simulink model "QDrone_IO_Check_Full_r2018a"  (Simulink 9.1)
settings: Solver=ode2  StartTime=0.0  StopTime=inf  FixedStep=0.001  RelTol=1e-3  EnableMultiTasking=on
model workspace (MAT data in the model file):
  Sig = Simulink.Signal
  Sig.DataType = 'auto'
  Sig.Dimensions = -1
  Sig.DimensionsMode = 'auto'
  Sig.Complexity = 'auto'
  Sig.SampleTime = -1
  Sig.SamplingMode = 'auto'
  video_step_size = 0.06
InitFcn:
  | set_param('QDrone_IO_Check_Full/Motor Switch', 'sw', '0');
undefined symbols (not defined in the file): HIL, qc_get_step_size
libraries: quarc_library x26, simulink x8, simulink_extras x3
settings Model: Creator=Admin  LastModifiedBy=user  SimulationMode=external
settings SolverCC: PositivePriorityOrder=on
settings DataIOCC: SaveFormat=Dataset
settings OptimizationCC: LifeSpan=auto
settings DebuggingCC: UnderspecifiedInitializationDetection=Simplified  MergeDetectMultiDrivingBlocksExec=error  ParameterPrecisionLossMsg=none
settings HardwareCC: ProdBitPerLong=64  ProdBitPerPointer=64  ProdBitPerSizeT=64  ProdBitPerPtrDiffT=64  ProdLargestAtomicFloat=Float  ProdIntDivRoundTo=Zero  ProdEndianess=LittleEndian  ProdWordSize=64  ProdHWDeviceType=Intel->x86-64 (Linux 64)
settings ModelReferenceCC: PropagateSignalLabelsOutOfModel=on
settings RTWCC: Description=QUARC Linux x64 Target (QDrone) Using Toolchain  SystemTargetFile=quarc_linux_x64.tlc  TemplateMakefile=quarc_default_tmf  Toolchain=QUARC linux_x64 | gmake (64-bit Windows)  BuildConfiguration=Faster Runs
settings STFCustomTargetCC: ConcurrentExecutionCompliant=on  UseToolchainInfoCompliant=on  SystemTargetFile=quarc_linux_x64.tlc
settings GRTTargetCC: ParMdlRefBuildCompliant=off  CompOptLevelCompliant=off  MatFileLogging=off  CPPClassGenCompliant=off  ExtMode=on  ExtModeMexFile=quarc_comm  ExtModeMexArgs='-w -d /tmp -uri %u','tcpip://QDrone0xxxxx.local:17001'

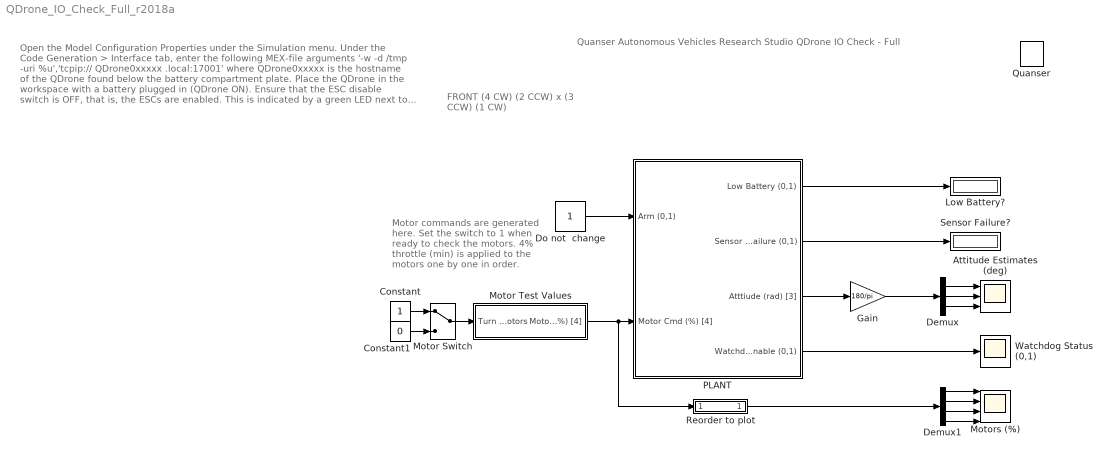
== system QDrone_IO_Check_Full_r2018a ==
  note: FRONT
      |
      | (4 CW)           (2 CCW)
      |
      |                 x
      |
      | (3 CCW)        (1 CW)
  note: Motor commands are generated here.
      |
      | Set the switch to 1 when ready to check
      | the motors. 4% throttle (min) is applied
      | to the motors one by one in order.
  note: Quanser Autonomous Vehicles Research Studio
      | QDrone IO Check - Full
  note: Open the Model Configuration Properties under the Simulation menu.
      |
      | Under the Code Generation > Interface tab, enter the following MEX-file arguments
      |
      | '-w -d /tmp -uri %u','tcpip:// QDrone0xxxxx .local:17001'
      |
      | where QDrone0xxxxx is the hostname of the QDrone found below the battery compartment plate.
      |
      | Place the QDrone in the workspace with a battery plugged in (QDrone ON).
      |
      | Ensure that the ESC disable switch is OFF, that is, the ESCs are enabled. This is indicated by a green LED next to the switch.
      |
      | Ensure that a connection to the drone is established by pinging to it. See the Research Studio Setup documentation (the Communicating with the QDrone section).
      |
      | Under the QUARC menu, click on Build .
      |
      | Ensure that the Motor Switch is set to 0 in this model.
      |
      | Under the QUARC menu, click on Start .
      |
      | After you hear 2 beeps (which indicates that the model has started running on the QDrone and that the ESCs are ENABLED), set the Motor Switch to 1.
      |
      | Ensure that the motors are spinning in order and directions specified in the Motors scope (they should turn on in the order of a clockwise circle).
      |
      | Set the Motor Switch to 0. Enter the workspace and set the ESC disable switch ON. This is indicated by a red LED next to the switch.
      |
      | Move the drone manually. Check the attitude of the drone in the Attitude Estimates (deg) scope to ensure that the readings are reasonable.
      | NOTE : Hold the drone using the handle on the top frame of the drone
      | NOTE : DO NOT handle the drone with spinning motors.
      | NOTE : Ensure that the motors are not spinning (Motor Switch set to 0). It is dangerous to handle the drone with spinning motors.
      |
      | Ensure that the Low Battery display shows 0 (as in your new Battery is not low. The low battery threshold is set to 10.5V)
      |
      | Ensure that the Sensor display shows 0 (no sensor failure detected).
  Attitude Estimates (deg) : Scope  NumInputPorts=3
  Constant : Constant
  Constant1 : Constant  Value=0
  Demux : Demux  Outputs=3
  Demux1 : Demux
  Do not  change : Constant
  Gain : Gain  Gain=180/pi
  Low Battery? : Display
      settings: Decimation=100
  Motor Switch : ManualSwitch
  Motor Test Values : Subsystem
  Motors (%) : Scope  NumInputPorts=4
  PLANT : Subsystem
  Quanser : quarc_library/Logos/Quanser
  Reorder to plot : Subsystem
  Sensor Failure? : Display
      settings: Decimation=100
  Watchdog Status (0,1) : Scope
  wires:
  PLANT/3(Atttiude (rad) [3]) -> Gain/1
  Constant/1 -> Motor Switch/1
  Constant1/1 -> Motor Switch/2
  Motor Test Values/1(Motor Cmd (%) [4]) -> Reorder to plot/1(" "), PLANT/2(Motor Cmd (%) [4])
  Demux1/1 -> Motors (%)/1
  Demux1/2 -> Motors (%)/2
  Demux1/3 -> Motors (%)/3
  Demux1/4 -> Motors (%)/4
  Demux/1 -> Attitude Estimates (deg)/1
  Demux/2 -> Attitude Estimates (deg)/2
  Demux/3 -> Attitude Estimates (deg)/3
  Motor Switch/1 -> Motor Test Values/1(Turn Motors)
  Gain/1 -> Demux/1
  Reorder to plot/1("  ") -> Demux1/1
  PLANT/2(Sensor Failure (0,1)) -> Sensor Failure?/1
  Do not  change/1 -> PLANT/1(Arm (0,1))
  PLANT/1(Low Battery (0,1)) -> Low Battery?/1
  PLANT/4(Watchdog Enable (0,1)) -> Watchdog Status (0,1)/1

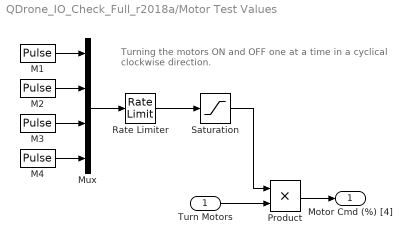
== system QDrone_IO_Check_Full_r2018a/Motor Test Values ==
  note: Turning the motors ON and OFF one at a time in a cyclical
      | clockwise direction.
  Turn Motors : Inport
  M1 : DiscretePulseGenerator  PulseType=Time based  Amplitude=0.04  Period=8  PulseWidth=12.5
  M2 : DiscretePulseGenerator  PulseType=Time based  Amplitude=0.04  Period=8  PulseWidth=12.5  PhaseDelay=6
  M3 : DiscretePulseGenerator  PulseType=Time based  Amplitude=0.04  Period=8  PulseWidth=12.5  PhaseDelay=2
  M4 : DiscretePulseGenerator  PulseType=Time based  Amplitude=0.04  Period=8  PulseWidth=12.5  PhaseDelay=4
  Mux : Mux
  Product : Product
  Rate Limiter : RateLimiter  RisingSlewLimit=0.1  FallingSlewLimit=-0.1  SampleTimeMode=inherited
  Saturation : Saturate  UpperLimit=0.1  LowerLimit=0
  Motor Cmd (%) [4] : Outport  VectorParamsAs1DForOutWhenUnconnected=off
  wires:
  M2/1 -> Mux/2
  M3/1 -> Mux/3
  M4/1 -> Mux/4
  M1/1 -> Mux/1
  Mux/1 -> Rate Limiter/1
  Rate Limiter/1 -> Saturation/1
  Saturation/1 -> Product/1
  Product/1 -> Motor Cmd (%) [4]/1
  Turn Motors/1 -> Product/2

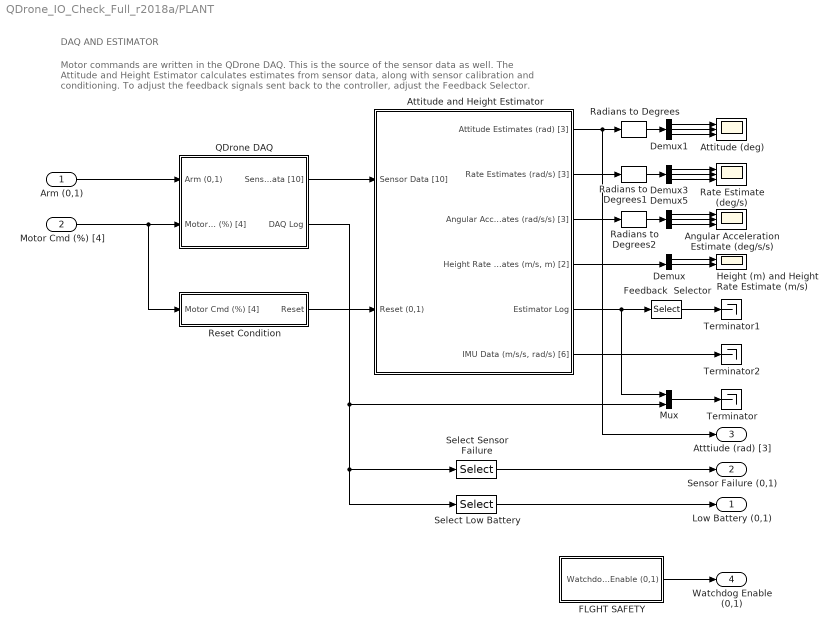
== system QDrone_IO_Check_Full_r2018a/PLANT ==
  note: Motor commands are written in the QDrone DAQ. This is the source of the sensor data as well. The Attitude and Height Estimator calculates estimates from sensor data, along with sensor calibration and conditioning. To adjust the feedback signals sent back to the controller, adjust the Feedback Selector.
  note: DAQ AND ESTIMATOR
  Arm (0,1) : Inport
  Motor Cmd (%) [4] : Inport  Port=2
  Angular Acceleration Estimate (deg/s/s) : Scope  NumInputPorts=3
  Attitude (deg) : Scope  NumInputPorts=3
  Attitude and Height Estimator : Subsystem
  Demux : Demux  Outputs=2
  Demux1 : Demux  Outputs=3
  Demux3 : Demux  Outputs=3
  Demux5 : Demux  Outputs=3
  FLGHT SAFETY : Subsystem
  Feedback  Selector : Selector  InputPortWidth=11  IndexOptions=Index vector (dialog)  Indices=[1:9]  OutputSizes=1
  Height (m) and Height Rate Estimate (m/s) : Scope  NumInputPorts=2
  Mux : Mux  Inputs=[11 13]
  QDrone DAQ : Subsystem
  Radians to Degrees : simulink_extras/Transformations/Radians to Degrees
  Radians to Degrees1 : simulink_extras/Transformations/Radians to Degrees
  Radians to Degrees2 : simulink_extras/Transformations/Radians to Degrees
  Rate Estimate (deg/s) : Scope  NumInputPorts=3
  Reset Condition : Subsystem
  Select Low Battery : Selector  InputPortWidth=13  IndexOptions=Index vector (dialog)  Indices=[3]  OutputSizes=1
  Select Sensor Failure : Selector  InputPortWidth=13  IndexOptions=Index vector (dialog)  Indices=[1]  OutputSizes=1
  Terminator : Terminator
  Terminator1 : Terminator
  Terminator2 : Terminator
  Low Battery (0,1) : Outport  VectorParamsAs1DForOutWhenUnconnected=off
  Sensor Failure (0,1) : Outport  Port=2  VectorParamsAs1DForOutWhenUnconnected=off
  Atttiude (rad) [3] : Outport  Port=3  VectorParamsAs1DForOutWhenUnconnected=off
  Watchdog Enable (0,1) : Outport  Port=4  VectorParamsAs1DForOutWhenUnconnected=off
  wires:
  Mux/1 -> Terminator/1
  QDrone DAQ/1(Sensor Data [10]) -> Attitude and Height Estimator/1(Sensor Data [10])
  Attitude and Height Estimator/4("Height Rate and  Height Estimates (m/s, m) [2]") -> Demux/1
  Attitude and Height Estimator/1(Attitude Estimates (rad) [3]) -> Atttiude (rad) [3]/1, Radians to Degrees/1
  Demux1/1 -> Attitude (deg)/1
  Demux1/2 -> Attitude (deg)/2
  Demux1/3 -> Attitude (deg)/3
  Demux3/1 -> Rate Estimate (deg/s)/1
  Demux3/2 -> Rate Estimate (deg/s)/2
  Demux3/3 -> Rate Estimate (deg/s)/3
  Demux5/1 -> Angular Acceleration Estimate (deg/s/s)/1
  Demux5/2 -> Angular Acceleration Estimate (deg/s/s)/2
  Demux5/3 -> Angular Acceleration Estimate (deg/s/s)/3
  Attitude and Height Estimator/2(Rate Estimates (rad/s) [3]) -> Radians to Degrees1/1
  Attitude and Height Estimator/3(Angular Acceleration Estimates (rad/s/s) [3]) -> Radians to Degrees2/1
  Demux/2 -> Height (m) and Height Rate Estimate (m/s)/2
  Demux/1 -> Height (m) and Height Rate Estimate (m/s)/1
  Attitude and Height Estimator/5(Estimator Log) -> Feedback  Selector/1, Mux/1
  Reset Condition/1(Reset) -> Attitude and Height Estimator/2(Reset (0,1))
  Motor Cmd (%) [4]/1 -> QDrone DAQ/2(Motor Cmd (%) [4]), Reset Condition/1(Motor Cmd (%) [4])
  Arm (0,1)/1 -> QDrone DAQ/1(Arm (0,1))
  Feedback  Selector/1 -> Terminator1/1
  QDrone DAQ/2(DAQ Log) -> Select Sensor Failure/1, Select Low Battery/1, Mux/2
  Select Low Battery/1 -> Low Battery (0,1)/1
  Select Sensor Failure/1 -> Sensor Failure (0,1)/1
  Attitude and Height Estimator/6("IMU Data (m/s/s, rad/s) [6]") -> Terminator2/1
  Radians to Degrees/1 -> Demux1/1
  Radians to Degrees1/1 -> Demux3/1
  Radians to Degrees2/1 -> Demux5/1
  FLGHT SAFETY/1(Watchdog Enable (0,1)) -> Watchdog Enable (0,1)/1

== system QDrone_IO_Check_Full_r2018a/Reorder to plot ==
  " " : Inport
  Demux : Demux
  Mux : Mux
  "  " : Outport  VectorParamsAs1DForOutWhenUnconnected=off
  wires:
  Demux/3 -> Mux/2
  Demux/4 -> Mux/1
  Mux/1 -> "  "/1
  Demux/2 -> Mux/3
  Demux/1 -> Mux/4
  " "/1 -> Demux/1

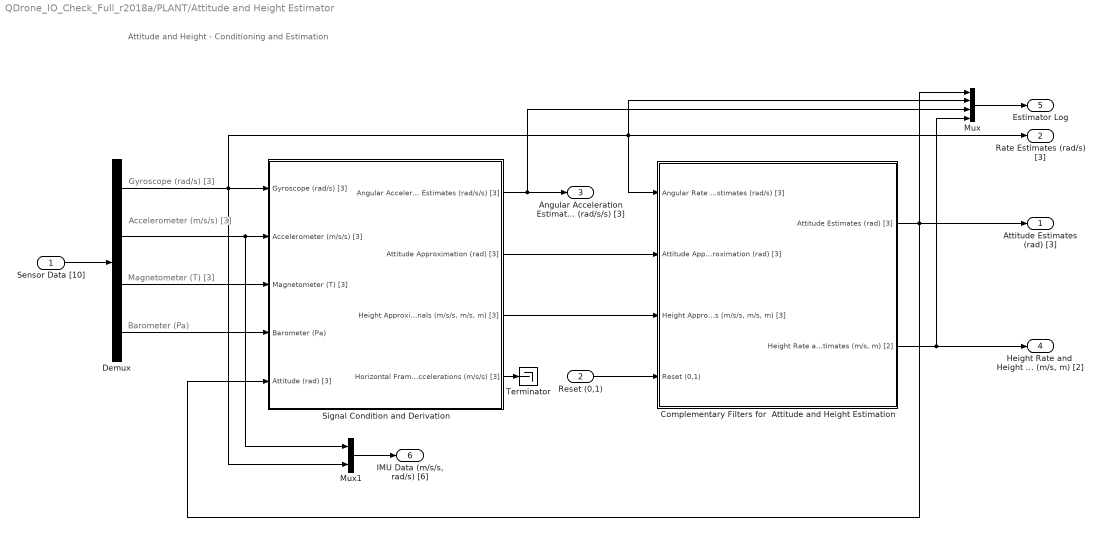
== system QDrone_IO_Check_Full_r2018a/PLANT/Attitude and Height Estimator ==
  note: Attitude and Height - Conditioning and Estimation
  note: Gyroscope (rad/s) [3]
  note: Accelerometer (m/s/s) [3]
  note: Magnetometer (T) [3]
  note: Barometer (Pa)
  Sensor Data [10] : Inport
  Reset (0,1) : Inport  Port=2
  Complementary Filters for  Attitude and Height Estimation : Subsystem
  Demux : Demux  Outputs=[3 3 3 1]
  Mux : Mux  Inputs=[3 3 3 2]
  Mux1 : Mux  Inputs=2
  Signal Condition and Derivation : Subsystem
  Terminator : Terminator
  Attitude Estimates (rad) [3] : Outport  VectorParamsAs1DForOutWhenUnconnected=off
  Rate Estimates (rad/s) [3] : Outport  Port=2  VectorParamsAs1DForOutWhenUnconnected=off
  Angular Acceleration Estimates (rad/s/s) [3] : Outport  Port=3  VectorParamsAs1DForOutWhenUnconnected=off
  "Height Rate and  Height Estimates (m/s, m) [2]" : Outport  Port=4  VectorParamsAs1DForOutWhenUnconnected=off
  Estimator Log : Outport  Port=5  VectorParamsAs1DForOutWhenUnconnected=off
  "IMU Data (m/s/s, rad/s) [6]" : Outport  Port=6  VectorParamsAs1DForOutWhenUnconnected=off
  wires:
  Complementary Filters for  Attitude and Height Estimation/2("Height Rate and  Height Estimates (m/s, m) [2]") -> "Height Rate and  Height Estimates (m/s, m) [2]"/1, Mux/4
  Signal Condition and Derivation/2(Attitude Approximation (rad) [3]) -> Complementary Filters for  Attitude and Height Estimation/2(Attitude Approximation (rad) [3])
  Signal Condition and Derivation/3("Height Approximation Signals (m/s/s, m/s, m) [3]") -> Complementary Filters for  Attitude and Height Estimation/3("Height Approximation Signals (m/s/s, m/s, m) [3]")
  Demux/2 -> Mux1/1, Signal Condition and Derivation/2(Accelerometer (m/s/s) [3])
  Demux/3 -> Signal Condition and Derivation/3(Magnetometer (T) [3])
  Demux/4 -> Signal Condition and Derivation/4(Barometer (Pa))
  Sensor Data [10]/1 -> Demux/1
  Mux/1 -> Estimator Log/1
  Reset (0,1)/1 -> Complementary Filters for  Attitude and Height Estimation/4(Reset (0,1))
  Complementary Filters for  Attitude and Height Estimation/1(Attitude Estimates (rad) [3]) -> Attitude Estimates (rad) [3]/1, Signal Condition and Derivation/5(Attitude (rad) [3]), Mux/1
  Signal Condition and Derivation/1(Angular Acceleration Estimates (rad/s/s) [3]) -> Mux/3, Angular Acceleration Estimates (rad/s/s) [3]/1
  Demux/1 -> Rate Estimates (rad/s) [3]/1, Mux/2, Complementary Filters for  Attitude and Height Estimation/1(Angular Rate Estimates (rad/s) [3]), Mux1/2, Signal Condition and Derivation/1(Gyroscope (rad/s) [3])
  Mux1/1 -> "IMU Data (m/s/s, rad/s) [6]"/1
  Signal Condition and Derivation/4(Horizontal Frame Accelerations (m/s/s) [3]) -> Terminator/1

== system QDrone_IO_Check_Full_r2018a/PLANT/FLGHT SAFETY ==
  note: Show if the watchdog is enabled/disabled via ESC enable switch.
  Data Type Conversion : DataTypeConversion  OutDataTypeStr=boolean
  HIL Watchdog : quarc_library/Data Acquisition/Generic/Watchdog/HIL Watchdog  object_name=HIL-1  timeout=0.1  sample_time=qc_get_step_size  active=off
      settings: AttributesFormatString=(%<object_name>)  SourceProductName=QUARC Targets
  Watchdog Enable (0,1) : Outport  VectorParamsAs1DForOutWhenUnconnected=off
  wires:
  HIL Watchdog/1 -> Data Type Conversion/1
  Data Type Conversion/1 -> Watchdog Enable (0,1)/1

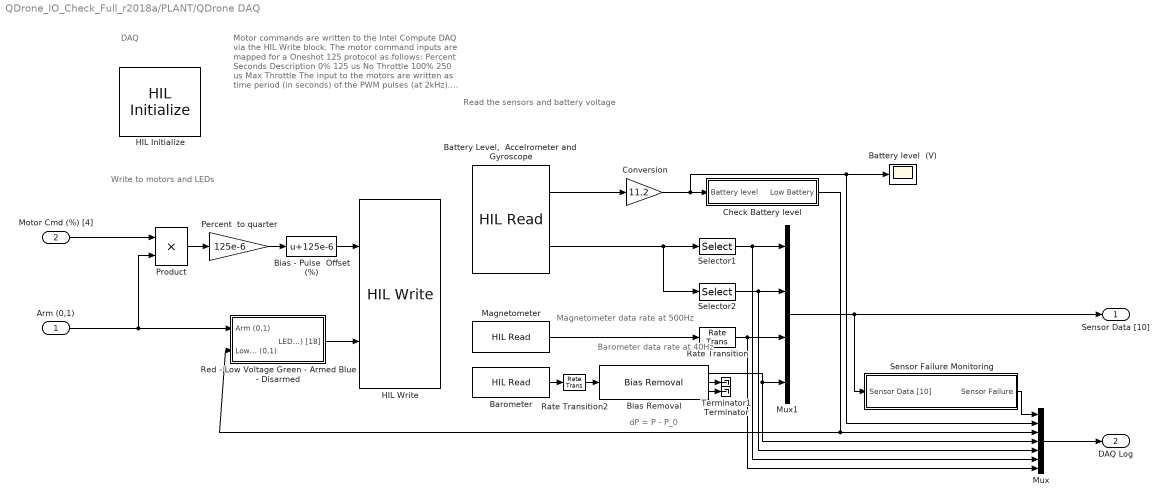
== system QDrone_IO_Check_Full_r2018a/PLANT/QDrone DAQ ==
  note: Read the sensors and battery voltage
  note: Write to motors and LEDs
  note: DAQ
  note: Motor commands are written to the Intel Compute DAQ via the HIL Write block. The motor command inputs are mapped for a Oneshot 125 protocol as follows:
      |
      | Percent Seconds Description
      | 0% 125 us No Throttle
      | 100% 250 us Max Throttle
      |
      | The input to the motors are written as time period (in seconds) of the PWM pulses (at 2kHz).
      |
      | LED colors can be set using a simple 3x1 ON (1) and OFF (0) vector (RGB mode).
  note: Barometer data rate at 40Hz
  note: Magnetometer data rate at 500Hz
  note: dP = P - P_0
  Arm (0,1) : Inport
  Motor Cmd (%) [4] : Inport  Port=2
  Barometer : quarc_library/Data Acquisition/Generic/Immediate I//O/HIL Read  Priority=1  object_name=HIL-1  analog_channels=[]  encoder_channels=[]  digital_channels=[]  other_channels=[9000]  sample_time=qc_get_step_size*25  active=on  vector_output=on  data_type_mode=Inherit via back propagation  encoder_data_type=double  digital_data_type=boolean
      settings: SourceProductName=The database C:\Users\user\AppData\Roaming\MathWorks\MATLAB\R2017a\slblocks_master.db is locked, or a table in the database is locked. (database is locked)
  "Battery Level,  Accelrometer and  Gyroscope" : quarc_library/Data Acquisition/Generic/Immediate I//O/HIL Read  Priority=1  object_name=HIL-1  analog_channels=[4]  encoder_channels=[]  digital_channels=[]  other_channels=[3000:3002 4000:4002]  sample_time=qc_get_step_size  active=on  vector_output=on  data_type_mode=Inherit via back propagation  encoder_data_type=double  digital_data_type=boolean
      settings: SourceProductName=The database C:\Users\user\AppData\Roaming\MathWorks\MATLAB\R2017a\slblocks_master.db is locked, or a table in the database is locked. (database is locked)
  Battery level  (V) : Scope
  Bias - Pulse  Offset (%) : Bias  Bias=125e-6
  Bias Removal : quarc_library/Discrete/Bias Removal  start_time=0  end_time=2  switch_id=X  sample_time=qc_get_step_size
      settings: SourceProductName=QUARC Targets
  Check Battery level : Subsystem
  Conversion : Gain  Gain=11.2
  HIL Initialize : quarc_library/Data Acquisition/Generic/Configuration/HIL Initialize  object_name=HIL-1  board_type=qdrone  board_number=0  board_options=gyro_fs=2000;gyro_rate=1000;gyro_os=4;accel_fs=16;accel_rate=400;accel_os=4;baro_os=4096  exclusive=off  active=on  hardware_clocks=[]  clock_modes=[]  initial_clock_frequencies=[]  set_clock_params_at_start=off  set_clock_params_at_switch_in=off  set_clock_frequencies_at_start=off  set_clock_frequencies_at_switch_in=off  analog_input_channels=[0:4]  analog_input_configurations=[]  analog_input_maximums=[3.3]  analog_input_minimums=[0]  set_analog_input_params_at_start=off  set_analog_input_params_at_switch_in=off  analog_output_channels=[]  analog_output_maximums=[]  analog_output_minimums=[]  initial_analog_outputs=[]  final_analog_outputs=[]  watchdog_analog_outputs=[]  set_analog_output_params_at_start=off  set_analog_output_params_at_switch_in=off  set_analog_outputs_at_start=off  set_analog_outputs_at_switch_in=off  set_analog_outputs_at_terminate=off  set_analog_outputs_at_switch_out=off  set_analog_outputs_on_watchdog=off  digital_input_channels=[]  digital_output_channels=[5:7 9:23]  digital_output_configuration=[]  initial_digital_outputs=[0]  final_digital_outputs=[0]  watchdog_digital_outputs=[]  set_digital_output_params_at_start=off  set_digital_output_params_at_switch_in=off  set_digital_outputs_at_start=on  set_digital_outputs_at_switch_in=off  set_digital_outputs_at_terminate=on  set_digital_outputs_at_switch_out=off  set_digital_outputs_on_watchdog=off  encoder_channels=[0:2]  quadrature=[4]  encoder_filter_frequency=50e6/1  initial_encoder_counts=[0]  set_encoder_params_at_start=on  set_encoder_params_at_switch_in=off  set_encoder_counts_at_start=on  set_encoder_counts_at_switch_in=off  pwm_channels=[0:3]  pwm_modes=[4]  pwm_frequency=2000  pwm_configuration=[0]  pwm_alignment=[0]  pwm_polarity=[1]  pwm_leading_deadband=[]  pwm_trailing_deadband=[]  initial_pwm_outputs=[0]  final_pwm_outputs=[0]  watchdog_pwm_outputs=[0]  set_pwm_params_at_start=on  set_pwm_params_at_switch_in=off  set_pwm_outputs_at_start=on  set_pwm_outputs_at_switch_in=off  set_pwm_outputs_at_terminate=on  set_pwm_outputs_at_switch_out=off  set_pwm_outputs_on_watchdog=off  other_output_channels=[]  initial_other_outputs=[]  final_other_outputs=[]  watchdog_other_outputs=[]  set_other_outputs_at_start=off  set_other_outputs_at_switch_in=off  set_other_outputs_at_terminate=off  set_other_outputs_at_switch_out=off  set_other_outputs_on_watchdog=off
      settings: SourceProductName=The database C:\Users\user\AppData\Roaming\MathWorks\MATLAB\R2017a\slblocks_master.db is locked, or a table in the database is locked. (database is locked)
  HIL Write : quarc_library/Data Acquisition/Generic/Immediate I//O/HIL Write  object_name=HIL-1  analog_channels=[]  pwm_channels=[0:3]  digital_channels=[5:7 9:23]  other_channels=[]  sample_time=-1  active=off  vector_input=on
      settings: SourceProductName=The database C:\Users\user\AppData\Roaming\MathWorks\MATLAB\R2017a\slblocks_master.db is locked, or a table in the database is locked. (database is locked)
  Magnetometer : quarc_library/Data Acquisition/Generic/Immediate I//O/HIL Read  Priority=1  object_name=HIL-1  analog_channels=[]  encoder_channels=[]  digital_channels=[]  other_channels=[8000:8002]  sample_time=qc_get_step_size*2  active=on  vector_output=on  data_type_mode=Inherit via back propagation  encoder_data_type=double  digital_data_type=boolean
      settings: SourceProductName=The database C:\Users\user\AppData\Roaming\MathWorks\MATLAB\R2017a\slblocks_master.db is locked, or a table in the database is locked. (database is locked)
  Mux : Mux  Inputs=[1 1 1 1 3 3 3]
  Mux1 : Mux  Inputs=[3 3 3 1]
  Percent  to quarter : Gain  Gain=125e-6
  Product : Product
  Rate Transition : RateTransition
  Rate Transition2 : RateTransition  OutPortSampleTime=qc_get_step_size
  Red - Low Voltage Green - Armed Blue - Disarmed : Subsystem
  Selector1 : Selector  InputPortWidth=6  IndexOptions=Index vector (dialog)  Indices=[1:3]  OutputSizes=1
  Selector2 : Selector  InputPortWidth=6  IndexOptions=Index vector (dialog)  Indices=[4:6]  OutputSizes=1
  Sensor Failure Monitoring : Subsystem
  Terminator : Terminator
  Terminator1 : Terminator
  Sensor Data [10] : Outport  VectorParamsAs1DForOutWhenUnconnected=off
  DAQ Log : Outport  Port=2  VectorParamsAs1DForOutWhenUnconnected=off
  wires:
  Percent  to quarter/1 -> Bias - Pulse  Offset (%)/1
  Arm (0,1)/1 -> Product/2, Red - Low Voltage Green - Armed Blue - Disarmed/1(Arm (0,1))
  "Battery Level,  Accelrometer and  Gyroscope"/2 -> Selector2/1, Selector1/1
  Check Battery level/1(Low Battery) -> Mux/3, Red - Low Voltage Green - Armed Blue - Disarmed/2(Low Battery (0,1))
  Sensor Failure Monitoring/1(Sensor Failure) -> Mux/1
  Magnetometer/1 -> Rate Transition/1
  Mux/1 -> DAQ Log/1
  Bias Removal/1 -> Mux/4, Mux1/4
  Selector2/1 -> Mux/5, Mux1/2
  Selector1/1 -> Mux/6, Mux1/1
  Rate Transition/1 -> Mux/7, Mux1/3
  "Battery Level,  Accelrometer and  Gyroscope"/1 -> Conversion/1
  Mux1/1 -> Sensor Data [10]/1, Sensor Failure Monitoring/1(Sensor Data [10])
  Motor Cmd (%) [4]/1 -> Product/1
  Conversion/1 -> Battery level  (V)/1, Mux/2, Check Battery level/1(Battery level)
  Bias - Pulse  Offset (%)/1 -> HIL Write/1
  Red - Low Voltage Green - Armed Blue - Disarmed/1(LEDs (%) [18]) -> HIL Write/2
  Product/1 -> Percent  to quarter/1
  Bias Removal/3 -> Terminator/1
  Bias Removal/2 -> Terminator1/1
  Barometer/1 -> Rate Transition2/1
  Rate Transition2/1 -> Bias Removal/1

== system QDrone_IO_Check_Full_r2018a/PLANT/Reset Condition ==
  note: Detect motor start condition and reset estimators.
      | Default threshold is if motor commands are greater than minimum throttle (5% of max.) for over 0.2 seconds.
  Motor Cmd (%) [4] : Inport
  Compare : quarc_library/Logic Operations/Compare  operator=>  output_data_type=boolean
      settings: SourceProductName=QUARC Targets
  For some time continuously : quarc_library/Discontinuities/Threshold  operator=>=  param_src=Specify via dialog  threshold=0.5  duration=0.2
      settings: SourceProductName=QUARC Targets
  Logical Operator : Logic  Inputs=1  AllPortsSameDT=off  OutDataTypeStr=boolean
  Minimum Throttle (%) : Constant  Value=[0.05 0.05 0.05 0.05]
  Terminator4 : Terminator
  Reset : Outport  VectorParamsAs1DForOutWhenUnconnected=off
  wires:
  For some time continuously/1 -> Reset/1
  Motor Cmd (%) [4]/1 -> Compare/1
  For some time continuously/2 -> Terminator4/1
  Compare/1 -> Logical Operator/1
  Minimum Throttle (%)/1 -> Compare/2
  Logical Operator/1 -> For some time continuously/1

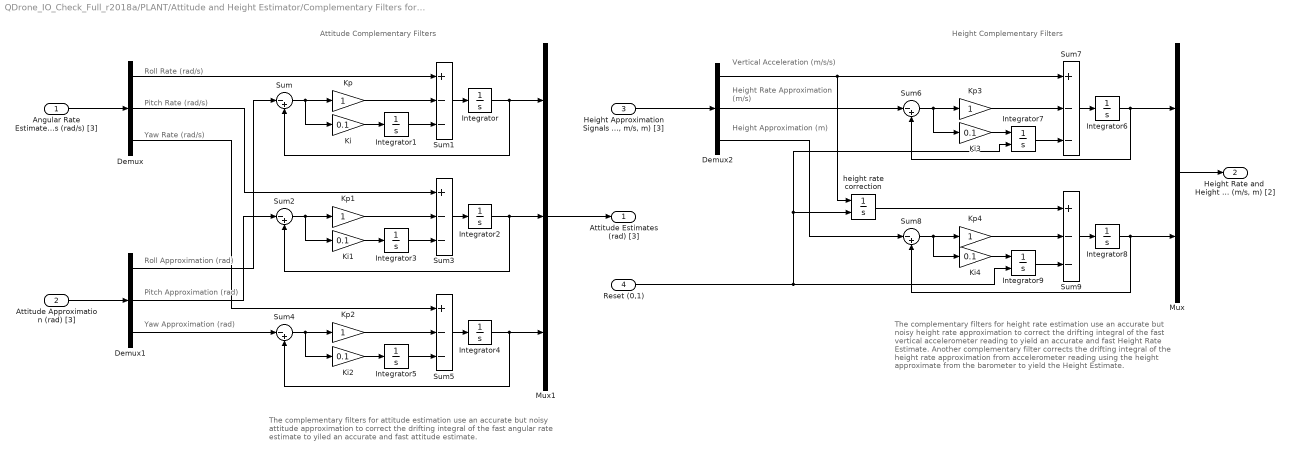
== system QDrone_IO_Check_Full_r2018a/PLANT/Attitude and Height Estimator/Complementary Filters for  Attitude and Height Estimation ==
  note: Attitude Complementary Filters
  note: The complementary filters for attitude estimation use an accurate but noisy attitude approximation to correct the drifting integral of the fast angular rate estimate to yiled an accurate and fast attitude estimate.
  note: Roll Rate (rad/s)
  note: Pitch Rate (rad/s)
  note: Yaw Rate (rad/s)
  note: Roll Approximation (rad)
  note: Pitch Approximation (rad)
  note: Yaw Approximation (rad)
  note: Height Rate Approximation (m/s)
  note: Height Approximation (m)
  note: Vertical Acceleration (m/s/s)
  note: Height Complementary Filters
  note: The complementary filters for height rate estimation use an accurate but noisy height rate approximation to correct the drifting integral of the fast vertical accelerometer reading to yield an accurate and fast Height Rate Estimate. Another complementary filter corrects the drifting integral of the height rate approximation from accelerometer reading using the height approximate from the barometer to yield the Height Estimate.
  Angular Rate Estimates (rad/s) [3] : Inport
  Attitude Approximation (rad) [3] : Inport  Port=2
  "Height Approximation Signals (m/s/s, m/s, m) [3]" : Inport  Port=3
  Reset (0,1) : Inport  Port=4
  Demux : Demux  Outputs=3
  Demux1 : Demux  Outputs=3
  Demux2 : Demux  Outputs=3
  Integrator{,1..6,8} (8 alike) : Integrator
  Integrator7 : Integrator  ExternalReset=rising
  Integrator9 : Integrator  ExternalReset=rising
  Ki{,1..4} (5 alike) : Gain  Gain=0.1
  Kp{,1..4} (5 alike) : Gain
  Mux : Mux  Inputs=2
  Mux1 : Mux  Inputs=3
  Sum{,2,4,6,8} (5 alike) : Sum  Inputs=|-+
  Sum{1,3,5,7,9} (5 alike) : Sum  Inputs=+--
  height rate correction : Integrator  ExternalReset=rising
  Attitude Estimates (rad) [3] : Outport  VectorParamsAs1DForOutWhenUnconnected=off
  "Height Rate and  Height Estimates (m/s, m) [2]" : Outport  Port=2  VectorParamsAs1DForOutWhenUnconnected=off
  wires:
  Integrator6/1 -> Sum6/2, Mux/1
  Angular Rate Estimates (rad/s) [3]/1 -> Demux/1
  Attitude Approximation (rad) [3]/1 -> Demux1/1
  Demux1/2 -> Sum2/1
  Demux1/3 -> Sum4/1
  Demux/2 -> Sum3/1
  Demux/3 -> Sum5/1
  Demux1/1 -> Sum/1
  Kp/1 -> Sum1/2
  Demux/1 -> Sum1/1
  Ki/1 -> Integrator1/1
  Integrator/1 -> Sum/2, Mux1/1
  Sum1/1 -> Integrator/1
  Integrator1/1 -> Sum1/3
  Sum/1 -> Ki/1, Kp/1
  Sum2/1 -> Kp1/1, Ki1/1
  Integrator3/1 -> Sum3/3
  Sum3/1 -> Integrator2/1
  Integrator2/1 -> Sum2/2, Mux1/2
  Ki1/1 -> Integrator3/1
  Kp1/1 -> Sum3/2
  Sum4/1 -> Kp2/1, Ki2/1
  Integrator5/1 -> Sum5/3
  Sum5/1 -> Integrator4/1
  Integrator4/1 -> Sum4/2, Mux1/3
  Ki2/1 -> Integrator5/1
  Kp2/1 -> Sum5/2
  Kp3/1 -> Sum7/2
  Ki3/1 -> Integrator7/1
  Sum7/1 -> Integrator6/1
  Integrator7/1 -> Sum7/3
  Sum6/1 -> Kp3/1, Ki3/1
  "Height Approximation Signals (m/s/s, m/s, m) [3]"/1 -> Demux2/1
  Demux2/1 -> Sum7/1, height rate correction/1
  Demux2/2 -> Sum6/1
  Sum8/1 -> Ki4/1, Kp4/1
  Integrator9/1 -> Sum9/3
  Sum9/1 -> Integrator8/1
  Ki4/1 -> Integrator9/1
  Kp4/1 -> Sum9/2
  Demux2/3 -> Sum8/1
  Integrator8/1 -> Sum8/2, Mux/2
  Reset (0,1)/1 -> Integrator9/2, Integrator7/2, height rate correction/2
  Mux/1 -> "Height Rate and  Height Estimates (m/s, m) [2]"/1
  height rate correction/1 -> Sum9/1
  Mux1/1 -> Attitude Estimates (rad) [3]/1

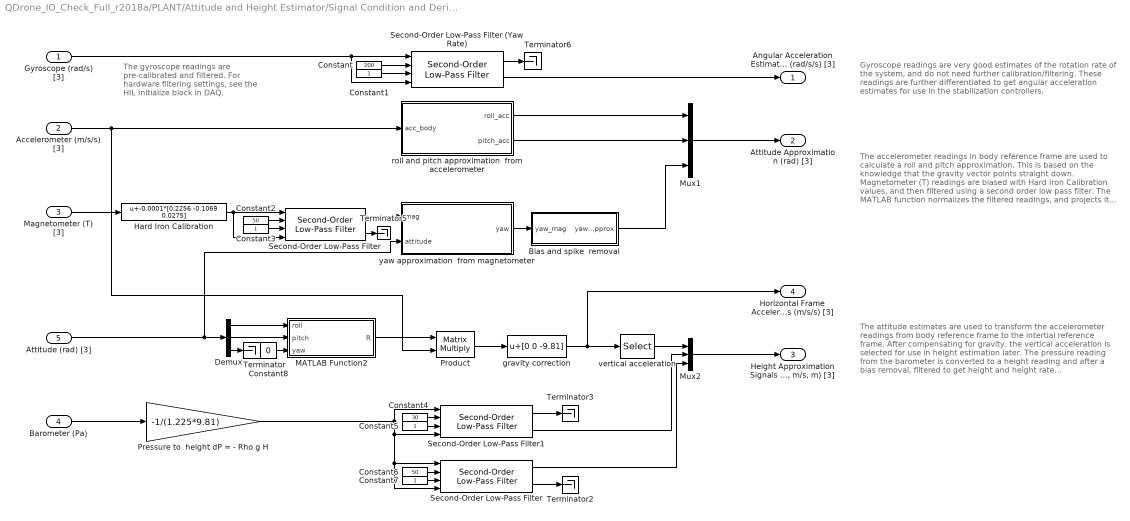
== system QDrone_IO_Check_Full_r2018a/PLANT/Attitude and Height Estimator/Signal Condition and Derivation ==
  note: The attitude estimates are used to transform the accelerometer readings from body reference frame to the intertial reference frame. After compensating for gravity, the vertical acceleration is selected for use in height estimation later.
      |
      | The pressure reading from the barometer is converted to a height reading and after a bias removal, filtered to get height and height rate approximations.
      |
      | The vertical acceleration, height rate approximation and height approximation are used in complementary filters to calculate height and height rate estimates.
  note: The accelerometer readings in body reference frame are used to calculate a roll and pitch approximation. This is based on the knowledge that the gravity vector points straight down. Magnetometer (T) readings are biased with Hard Iron Calibration values, and then filtered using a second order low pass filter. The MATLAB function normalizes the filtered readings, and projects it to the horizontal plane using the attitude estimates. This value is then biased with an initial reading to get a yaw approximation relative to the initial yaw.
  note: Gyroscope readings are very good estimates of the rotation rate of the system, and do not need further calibration/filtering. These readings are further differentiated to get angular acceleration estimates for use in the stabilization controllers.
  note: The gyroscope readings are pre-calibrated
      | and filtered. For hardware filtering settings,
      | see the HIL Initialize block in DAQ.
  Gyroscope (rad/s) [3] : Inport
  Accelerometer (m/s/s) [3] : Inport  Port=2
  Magnetometer (T) [3] : Inport  Port=3
  Barometer (Pa) : Inport  Port=4
  Attitude (rad) [3] : Inport  Port=5
  Bias and spike  removal : Subsystem
  Constant : Constant  Value=200
  Constant{1,3,5,7} (4 alike) : Constant
  Constant2 : Constant  Value=50
  Constant4 : Constant  Value=30
  Constant6 : Constant  Value=50
  Constant8 : Constant  Value=0
  Demux : Demux  Outputs=3
  Hard Iron Calibration : Bias  Bias=-0.0001*[0.2256 -0.1069 0.0275]
  MATLAB Function2 : MATLAB Function  TreatAsAtomicUnit=on
  Mux1 : Mux  Inputs=3
  Mux2 : Mux  Inputs=3
  Pressure to  height dP = - Rho g H : Gain  Gain=-1/(1.225*9.81)
  Product : Product  Multiplication=Matrix(*)
  Second-Order Low-Pass Filter : quarc_library/Continuous/Second-Order Low-Pass Filter  params_source=External (input ports)  input_width=50  input_zeta=1  input_init=0
      settings: SourceProductName=The database C:\Users\user\AppData\Roaming\MathWorks\MATLAB\R2017a\slblocks_master.db is locked, or a table in the database is locked. (database is locked)
  Second-Order Low-Pass Filter (Yaw Rate) : quarc_library/Continuous/Second-Order Low-Pass Filter  params_source=External (input ports)  input_width=200  input_zeta=1  input_init=0
      settings: SourceProductName=The database C:\Users\user\AppData\Roaming\MathWorks\MATLAB\R2017a\slblocks_master.db is locked, or a table in the database is locked. (database is locked)
  "Second-Order Low-Pass Filter " : quarc_library/Continuous/Second-Order Low-Pass Filter  params_source=External (input ports)  input_width=50  input_zeta=1  input_init=0
      settings: SourceProductName=The database C:\Users\user\AppData\Roaming\MathWorks\MATLAB\R2017a\slblocks_master.db is locked, or a table in the database is locked. (database is locked)
  Second-Order Low-Pass Filter1 : quarc_library/Continuous/Second-Order Low-Pass Filter  params_source=External (input ports)  input_width=30  input_zeta=1  input_init=0
      settings: SourceProductName=The database C:\Users\user\AppData\Roaming\MathWorks\MATLAB\R2017a\slblocks_master.db is locked, or a table in the database is locked. (database is locked)
  Terminator{,2..3,5..6} (5 alike) : Terminator
  gravity correction : Bias  Bias=[0 0 -9.81]
  roll and pitch approximation  from accelerometer : MATLAB Function  TreatAsAtomicUnit=on
  vertical acceleration : Selector  InputPortWidth=3  IndexOptions=Index vector (dialog)  Indices=[3]  OutputSizes=1
  yaw approximation  from magnetometer : MATLAB Function  TreatAsAtomicUnit=on
  Angular Acceleration Estimates (rad/s/s) [3] : Outport  VectorParamsAs1DForOutWhenUnconnected=off
  Attitude Approximation (rad) [3] : Outport  Port=2  VectorParamsAs1DForOutWhenUnconnected=off
  "Height Approximation Signals (m/s/s, m/s, m) [3]" : Outport  Port=3  VectorParamsAs1DForOutWhenUnconnected=off
  Horizontal Frame Accelerations (m/s/s) [3] : Outport  Port=4  VectorParamsAs1DForOutWhenUnconnected=off
  wires:
  Second-Order Low-Pass Filter1/1 -> Terminator3/1
  Pressure to  height dP = - Rho g H/1 -> Second-Order Low-Pass Filter/4, Second-Order Low-Pass Filter/1, Second-Order Low-Pass Filter1/4, Second-Order Low-Pass Filter1/1
  Accelerometer (m/s/s) [3]/1 -> roll and pitch approximation  from accelerometer/1(acc_body), Product/2
  Second-Order Low-Pass Filter/2 -> Terminator2/1
  Barometer (Pa)/1 -> Pressure to  height dP = - Rho g H/1
  MATLAB Function2/1(R) -> Product/1
  gravity correction/1 -> Horizontal Frame Accelerations (m/s/s) [3]/1, vertical acceleration/1
  Product/1 -> gravity correction/1
  "Second-Order Low-Pass Filter "/1 -> yaw approximation  from magnetometer/1(mag)
  Hard Iron Calibration/1 -> "Second-Order Low-Pass Filter "/4, "Second-Order Low-Pass Filter "/1
  Magnetometer (T) [3]/1 -> Hard Iron Calibration/1
  Second-Order Low-Pass Filter (Yaw Rate)/1 -> Terminator6/1
  yaw approximation  from magnetometer/1(yaw) -> Bias and spike  removal/1(yaw_mag)
  Gyroscope (rad/s) [3]/1 -> Second-Order Low-Pass Filter (Yaw Rate)/4, Second-Order Low-Pass Filter (Yaw Rate)/1
  "Second-Order Low-Pass Filter "/2 -> Terminator5/1
  roll and pitch approximation  from accelerometer/1(roll_acc) -> Mux1/1
  roll and pitch approximation  from accelerometer/2(pitch_acc) -> Mux1/2
  Bias and spike  removal/1(yaw_approx) -> Mux1/3
  Second-Order Low-Pass Filter/1 -> Mux2/3
  Second-Order Low-Pass Filter1/2 -> Mux2/2
  vertical acceleration/1 -> Mux2/1
  Mux2/1 -> "Height Approximation Signals (m/s/s, m/s, m) [3]"/1
  Attitude (rad) [3]/1 -> Demux/1, yaw approximation  from magnetometer/2(attitude)
  Mux1/1 -> Attitude Approximation (rad) [3]/1
  Second-Order Low-Pass Filter (Yaw Rate)/2 -> Angular Acceleration Estimates (rad/s/s) [3]/1
  Constant/1 -> Second-Order Low-Pass Filter (Yaw Rate)/2
  Constant1/1 -> Second-Order Low-Pass Filter (Yaw Rate)/3
  Constant2/1 -> "Second-Order Low-Pass Filter "/2
  Constant3/1 -> "Second-Order Low-Pass Filter "/3
  Constant4/1 -> Second-Order Low-Pass Filter1/2
  Constant6/1 -> Second-Order Low-Pass Filter/2
  Constant7/1 -> Second-Order Low-Pass Filter/3
  Constant5/1 -> Second-Order Low-Pass Filter1/3
  Demux/1 -> MATLAB Function2/1(roll)
  Demux/2 -> MATLAB Function2/2(pitch)
  Demux/3 -> Terminator/1
  Constant8/1 -> MATLAB Function2/3(yaw)

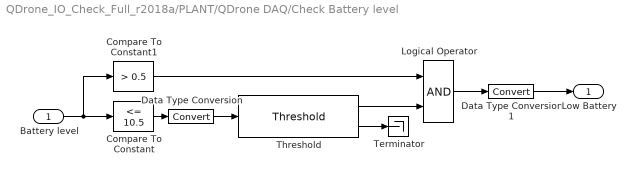
== system QDrone_IO_Check_Full_r2018a/PLANT/QDrone DAQ/Check Battery level ==
  Battery level : Inport
  Compare To Constant : simulink/Logic and Bit Operations/Compare To Constant  relop=<=  const=10.5  OutDataTypeStr=boolean
  Compare To Constant1 : simulink/Logic and Bit Operations/Compare To Constant  relop=>  const=0.5  OutDataTypeStr=boolean
  Data Type Conversion : DataTypeConversion
  Data Type Conversion1 : DataTypeConversion
  Logical Operator : Logic  AllPortsSameDT=off  OutDataTypeStr=boolean
  Terminator : Terminator
  Threshold : quarc_library/Discontinuities/Threshold  operator=>=  param_src=Specify via dialog  threshold=0.5  duration=0.1
      settings: SourceProductName=The database C:\Users\user\AppData\Roaming\MathWorks\MATLAB\R2017a\slblocks_master.db is locked, or a table in the database is locked. (database is locked)
  Low Battery : Outport  VectorParamsAs1DForOutWhenUnconnected=off
  wires:
  Threshold/2 -> Terminator/1
  Battery level/1 -> Compare To Constant1/1, Compare To Constant/1
  Threshold/1 -> Logical Operator/2
  Logical Operator/1 -> Data Type Conversion1/1
  Compare To Constant1/1 -> Logical Operator/1
  Compare To Constant/1 -> Data Type Conversion/1
  Data Type Conversion/1 -> Threshold/1
  Data Type Conversion1/1 -> Low Battery/1

== system QDrone_IO_Check_Full_r2018a/PLANT/QDrone DAQ/Red - Low Voltage Green - Armed Blue - Disarmed ==
  note: PCB LED 3
  note: PCB LED 2
  note: PCB LED 1
  note: PCB LED 5
  note: PCB LED 4
  note: Onboard LED
  Arm (0,1) : Inport
  Low Battery (0,1) : Inport  Port=2
  Blue : Constant  Value=[0 0 1]
  Green : Constant  Value=[0 1 0]
  MATLAB Function LED Color Assignment : MATLAB Function  TreatAsAtomicUnit=on
  Multiport Switch : MultiPortSwitch
  Mux : Mux  Inputs=[3 3 3 3 3 3]
  Red : Constant  Value=[1 0 0]
  LEDs (%) [18] : Outport  VectorParamsAs1DForOutWhenUnconnected=off
  wires:
  Multiport Switch/1 -> Mux/4, Mux/5, Mux/6, Mux/3, Mux/2, Mux/1
  Red/1 -> Multiport Switch/2
  Green/1 -> Multiport Switch/3
  Blue/1 -> Multiport Switch/4
  Arm (0,1)/1 -> MATLAB Function LED Color Assignment/1(arm)
  MATLAB Function LED Color Assignment/1(value) -> Multiport Switch/1
  Low Battery (0,1)/1 -> MATLAB Function LED Color Assignment/2(low_battery)
  Mux/1 -> LEDs (%) [18]/1

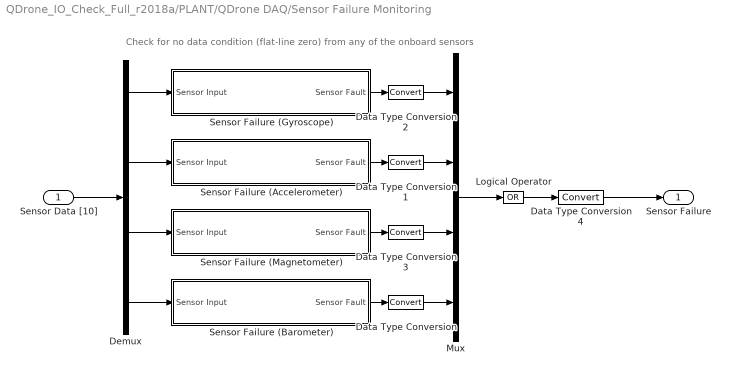
== system QDrone_IO_Check_Full_r2018a/PLANT/QDrone DAQ/Sensor Failure Monitoring ==
  note: Check for no data condition (flat-line zero) from any of the onboard sensors
  Sensor Data [10] : Inport
  Data Type Conversion{,1..4} (5 alike) : DataTypeConversion
  Demux : Demux  Outputs=[3 3 3 1]
  Logical Operator : Logic  Operator=OR  Inputs=1  AllPortsSameDT=off  OutDataTypeStr=boolean
  Mux : Mux
  Sensor Failure (Accelerometer) : Subsystem
  Sensor Failure (Barometer) : Subsystem
  Sensor Failure (Gyroscope) : Subsystem
  Sensor Failure (Magnetometer) : Subsystem
  Sensor Failure : Outport  VectorParamsAs1DForOutWhenUnconnected=off
  wires:
  Demux/2 -> Sensor Failure (Accelerometer)/1(Sensor Input)
  Sensor Failure (Barometer)/1(Sensor Fault) -> Data Type Conversion/1
  Sensor Failure (Gyroscope)/1(Sensor Fault) -> Data Type Conversion2/1
  Sensor Failure (Magnetometer)/1(Sensor Fault) -> Data Type Conversion3/1
  Sensor Failure (Accelerometer)/1(Sensor Fault) -> Data Type Conversion1/1
  Mux/1 -> Logical Operator/1
  Data Type Conversion2/1 -> Mux/1
  Data Type Conversion1/1 -> Mux/2
  Data Type Conversion3/1 -> Mux/3
  Data Type Conversion/1 -> Mux/4
  Sensor Data [10]/1 -> Demux/1
  Demux/1 -> Sensor Failure (Gyroscope)/1(Sensor Input)
  Demux/3 -> Sensor Failure (Magnetometer)/1(Sensor Input)
  Demux/4 -> Sensor Failure (Barometer)/1(Sensor Input)
  Logical Operator/1 -> Data Type Conversion4/1
  Data Type Conversion4/1 -> Sensor Failure/1

== system QDrone_IO_Check_Full_r2018a/PLANT/Attitude and Height Estimator/Signal Condition and Derivation/Bias and spike  removal ==
  note: Ignore the initial spike (before 0.1s). Subtract bias from the reading.
  yaw_mag : Inport
  Clock : Clock
  Compare To Constant : simulink/Logic and Bit Operations/Compare To Constant  relop=<=  const=1.0  OutDataTypeStr=boolean
  Compare To Constant1 : simulink/Logic and Bit Operations/Compare To Constant  relop=>=  const=0.1  OutDataTypeStr=boolean
  Initial Bias : Subsystem  TreatAsAtomicUnit=on
  Inverse Modulus1 : quarc_library/Discontinuities/Inverse Modulus  modulus=2*pi  output_derivative=off  output_revolutions=off  max_x=Inf  min_x=-Inf
      settings: SourceProductName=The database C:\Users\user\AppData\Roaming\MathWorks\MATLAB\R2017a\slblocks_master.db is locked, or a table in the database is locked. (database is locked)
  Remove Spike : Subsystem  TreatAsAtomicUnit=on
  Subtract : Sum  Inputs=-+
  yaw_approx : Outport  VectorParamsAs1DForOutWhenUnconnected=off
  wires:
  Compare To Constant/1 -> Initial Bias/Enable
  Compare To Constant1/1 -> Remove Spike/Enable
  Initial Bias/1(Yaw_0) -> Subtract/1
  Remove Spike/1("  ") -> yaw_approx/1
  Subtract/1 -> Remove Spike/1(" ")
  yaw_mag/1 -> Initial Bias/1(Yaw), Inverse Modulus1/1
  Inverse Modulus1/1 -> Subtract/2
  Clock/1 -> Compare To Constant1/1, Compare To Constant/1

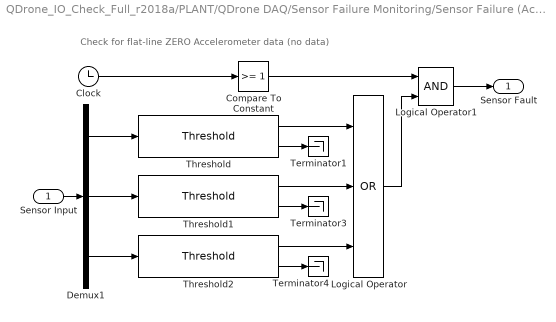
== system QDrone_IO_Check_Full_r2018a/PLANT/QDrone DAQ/Sensor Failure Monitoring/Sensor Failure (Accelerometer) ==
  note: Check for flat-line ZERO Accelerometer data (no data)
  Sensor Input : Inport
  Clock : Clock
  Compare To Constant : simulink/Logic and Bit Operations/Compare To Constant  relop=>=  const=1  OutDataTypeStr=boolean
  Demux1 : Demux  Outputs=3
  Logical Operator : Logic  Operator=OR  Inputs=3  AllPortsSameDT=off  OutDataTypeStr=boolean
  Logical Operator1 : Logic  AllPortsSameDT=off  OutDataTypeStr=boolean
  Terminator1 : Terminator
  Terminator3 : Terminator
  Terminator4 : Terminator
  Threshold : quarc_library/Discontinuities/Threshold  operator===  param_src=Specify via dialog  threshold=0  duration=1
      settings: SourceProductName=The database C:\Users\user\AppData\Roaming\MathWorks\MATLAB\R2017a\slblocks_master.db is locked, or a table in the database is locked. (database is locked)
  Threshold1 : quarc_library/Discontinuities/Threshold  operator===  param_src=Specify via dialog  threshold=0  duration=1
      settings: SourceProductName=The database C:\Users\user\AppData\Roaming\MathWorks\MATLAB\R2017a\slblocks_master.db is locked, or a table in the database is locked. (database is locked)
  Threshold2 : quarc_library/Discontinuities/Threshold  operator===  param_src=Specify via dialog  threshold=0  duration=1
      settings: SourceProductName=The database C:\Users\user\AppData\Roaming\MathWorks\MATLAB\R2017a\slblocks_master.db is locked, or a table in the database is locked. (database is locked)
  Sensor Fault : Outport  VectorParamsAs1DForOutWhenUnconnected=off
  wires:
  Threshold/2 -> Terminator1/1
  Threshold1/2 -> Terminator3/1
  Logical Operator/1 -> Logical Operator1/2
  Demux1/2 -> Threshold1/1
  Demux1/3 -> Threshold2/1
  Demux1/1 -> Threshold/1
  Threshold2/1 -> Logical Operator/3
  Threshold2/2 -> Terminator4/1
  Sensor Input/1 -> Demux1/1
  Logical Operator1/1 -> Sensor Fault/1
  Compare To Constant/1 -> Logical Operator1/1
  Threshold1/1 -> Logical Operator/2
  Threshold/1 -> Logical Operator/1
  Clock/1 -> Compare To Constant/1

== system QDrone_IO_Check_Full_r2018a/PLANT/QDrone DAQ/Sensor Failure Monitoring/Sensor Failure (Barometer) ==
  note: Check for flat-line ZERO Barometer data (no data)
  Sensor Input : Inport
  Clock : Clock
  Compare To Constant : simulink/Logic and Bit Operations/Compare To Constant  relop=>=  const=1  OutDataTypeStr=boolean
  Logical Operator1 : Logic  AllPortsSameDT=off  OutDataTypeStr=boolean
  Terminator1 : Terminator
  Threshold : quarc_library/Discontinuities/Threshold  operator===  param_src=Specify via dialog  threshold=0  duration=1
      settings: SourceProductName=The database C:\Users\user\AppData\Roaming\MathWorks\MATLAB\R2017a\slblocks_master.db is locked, or a table in the database is locked. (database is locked)
  Sensor Fault : Outport  VectorParamsAs1DForOutWhenUnconnected=off
  wires:
  Clock/1 -> Compare To Constant/1
  Compare To Constant/1 -> Logical Operator1/1
  Logical Operator1/1 -> Sensor Fault/1
  Sensor Input/1 -> Threshold/1
  Threshold/1 -> Logical Operator1/2
  Threshold/2 -> Terminator1/1

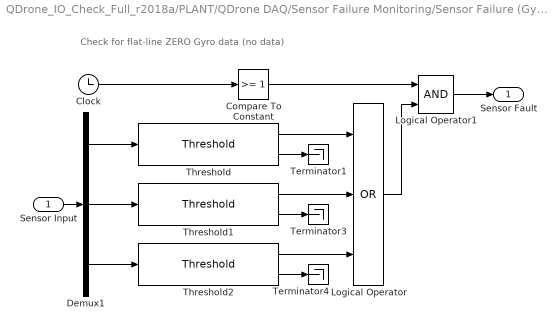
== system QDrone_IO_Check_Full_r2018a/PLANT/QDrone DAQ/Sensor Failure Monitoring/Sensor Failure (Gyroscope) ==
  note: Check for flat-line ZERO Gyro data (no data)
  Sensor Input : Inport
  Clock : Clock
  Compare To Constant : simulink/Logic and Bit Operations/Compare To Constant  relop=>=  const=1  OutDataTypeStr=boolean
  Demux1 : Demux  Outputs=3
  Logical Operator : Logic  Operator=OR  Inputs=3  AllPortsSameDT=off  OutDataTypeStr=boolean
  Logical Operator1 : Logic  AllPortsSameDT=off  OutDataTypeStr=boolean
  Terminator1 : Terminator
  Terminator3 : Terminator
  Terminator4 : Terminator
  Threshold : quarc_library/Discontinuities/Threshold  operator===  param_src=Specify via dialog  threshold=0  duration=1
      settings: SourceProductName=The database C:\Users\user\AppData\Roaming\MathWorks\MATLAB\R2017a\slblocks_master.db is locked, or a table in the database is locked. (database is locked)
  Threshold1 : quarc_library/Discontinuities/Threshold  operator===  param_src=Specify via dialog  threshold=0  duration=1
      settings: SourceProductName=The database C:\Users\user\AppData\Roaming\MathWorks\MATLAB\R2017a\slblocks_master.db is locked, or a table in the database is locked. (database is locked)
  Threshold2 : quarc_library/Discontinuities/Threshold  operator===  param_src=Specify via dialog  threshold=0  duration=1
      settings: SourceProductName=The database C:\Users\user\AppData\Roaming\MathWorks\MATLAB\R2017a\slblocks_master.db is locked, or a table in the database is locked. (database is locked)
  Sensor Fault : Outport  VectorParamsAs1DForOutWhenUnconnected=off
  wires:
  Clock/1 -> Compare To Constant/1
  Threshold/1 -> Logical Operator/1
  Threshold1/1 -> Logical Operator/2
  Compare To Constant/1 -> Logical Operator1/1
  Logical Operator1/1 -> Sensor Fault/1
  Sensor Input/1 -> Demux1/1
  Threshold2/2 -> Terminator4/1
  Threshold2/1 -> Logical Operator/3
  Demux1/1 -> Threshold/1
  Demux1/3 -> Threshold2/1
  Demux1/2 -> Threshold1/1
  Logical Operator/1 -> Logical Operator1/2
  Threshold1/2 -> Terminator3/1
  Threshold/2 -> Terminator1/1

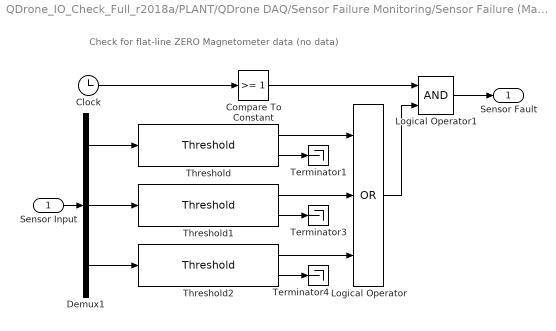
== system QDrone_IO_Check_Full_r2018a/PLANT/QDrone DAQ/Sensor Failure Monitoring/Sensor Failure (Magnetometer) ==
  note: Check for flat-line ZERO Magnetometer data (no data)
  Sensor Input : Inport
  Clock : Clock
  Compare To Constant : simulink/Logic and Bit Operations/Compare To Constant  relop=>=  const=1  OutDataTypeStr=boolean
  Demux1 : Demux  Outputs=3
  Logical Operator : Logic  Operator=OR  Inputs=3  AllPortsSameDT=off  OutDataTypeStr=boolean
  Logical Operator1 : Logic  AllPortsSameDT=off  OutDataTypeStr=boolean
  Terminator1 : Terminator
  Terminator3 : Terminator
  Terminator4 : Terminator
  Threshold : quarc_library/Discontinuities/Threshold  operator===  param_src=Specify via dialog  threshold=0  duration=1
      settings: SourceProductName=The database C:\Users\user\AppData\Roaming\MathWorks\MATLAB\R2017a\slblocks_master.db is locked, or a table in the database is locked. (database is locked)
  Threshold1 : quarc_library/Discontinuities/Threshold  operator===  param_src=Specify via dialog  threshold=0  duration=1
      settings: SourceProductName=The database C:\Users\user\AppData\Roaming\MathWorks\MATLAB\R2017a\slblocks_master.db is locked, or a table in the database is locked. (database is locked)
  Threshold2 : quarc_library/Discontinuities/Threshold  operator===  param_src=Specify via dialog  threshold=0  duration=1
      settings: SourceProductName=The database C:\Users\user\AppData\Roaming\MathWorks\MATLAB\R2017a\slblocks_master.db is locked, or a table in the database is locked. (database is locked)
  Sensor Fault : Outport  VectorParamsAs1DForOutWhenUnconnected=off
  wires:
  Threshold/2 -> Terminator1/1
  Threshold1/2 -> Terminator3/1
  Logical Operator/1 -> Logical Operator1/2
  Demux1/2 -> Threshold1/1
  Demux1/3 -> Threshold2/1
  Demux1/1 -> Threshold/1
  Threshold2/1 -> Logical Operator/3
  Threshold2/2 -> Terminator4/1
  Sensor Input/1 -> Demux1/1
  Logical Operator1/1 -> Sensor Fault/1
  Compare To Constant/1 -> Logical Operator1/1
  Threshold1/1 -> Logical Operator/2
  Threshold/1 -> Logical Operator/1
  Clock/1 -> Compare To Constant/1

== system QDrone_IO_Check_Full_r2018a/PLANT/Attitude and Height Estimator/Signal Condition and Derivation/Bias and spike  removal/Initial Bias ==
  Yaw : Inport
  Enable : EnablePort
  Yaw_0 : Outport  InitialOutput=[0]  VectorParamsAs1DForOutWhenUnconnected=off
  wires:
  Yaw/1 -> Yaw_0/1

== system QDrone_IO_Check_Full_r2018a/PLANT/Attitude and Height Estimator/Signal Condition and Derivation/Bias and spike  removal/Remove Spike ==
  " " : Inport
  Enable : EnablePort
  "  " : Outport  InitialOutput=[0]  VectorParamsAs1DForOutWhenUnconnected=off
  wires:
  " "/1 -> "  "/1

== matlab function PLANT/Attitude and Height Estimator/Signal Condition and Derivation/roll and pitch approximation from accelerometer ==
  data: roll_acc output double; pitch_acc output double; acc_body input double
function [roll_acc, pitch_acc]   = fcn(acc_body)
%#eml
n = norm(acc_body,2);
if n>eps
    acc_body = acc_body/n; 
else
    acc_body = [0 0 1]';
end

roll_acc = atan2(acc_body(2),acc_body(3));
pitch_acc = atan2( -acc_body(1), acc_body(2)*sin(roll_acc)+acc_body(3)*cos(roll_acc));

== matlab function PLANT/Attitude and Height Estimator/Signal Condition and Derivation/yaw approximation from magnetometer ==
  data: mag input double; yaw output double; attitude input double
function yaw = fcn(mag, attitude)
% attitude = [roll pitch yaw]';
mag_n = mag./(norm(mag, 2));
yaw = atan2(  mag_n(3)*sin(attitude(1)) - mag_n(2)*cos(attitude(1)) ,...
              mag_n(3)*cos(attitude(1))*sin(attitude(2)) + mag_n(2)*sin(attitude(1))*sin(attitude(2)) + mag_n(1)*cos(attitude(2)));

== matlab function PLANT/Attitude and Height Estimator/Signal Condition and Derivation/MATLAB Function2 ==
  data: roll input double; R output double; pitch input double; yaw input double
function R = rot_xyz(roll, pitch, yaw)

Rx  = [               1                 0           0        ;...
                      0  cos(roll)  -sin(roll) ;...
                      0  sin(roll)   cos(roll)];
       
Ry  = [cos(pitch)                 0   sin(pitch);...
                      0                 1                  0 ;...
       -sin(pitch)                 0   cos(pitch)];

Rz =  [cos(yaw) -sin(yaw)                  0 ;...
       sin(yaw)  cos(yaw)                  0 ;...
                      0                 0                  1];

R = Rx*Ry*Rz;

== matlab function PLANT/QDrone DAQ/Red - Low Voltage Green - Armed Blue - Disarmed/MATLAB Function LED Color Assignment ==
  data: arm input double; value output double; low_battery input double
function value = fcn(arm, low_battery)

if low_battery
    value = 1;
elseif arm
    value = 2;
else 
    value = 3;
end
